simulink model "UBR_SIMULINK_2"  (R2023a)
settings: Solver=VariableStepAuto  StartTime=0.0  StopTime=10  RelTol=1e-3
values from neighbouring files (symbols this model uses):
  g = 9.801    [ubr_3.m]
  vx0 = v0 * cos(theta0)    [ubr_3.m]
  vz0 = v0 * sin(theta0)    [ubr_3.m]
settings Model: Creator=sefab  LastModifiedBy=sefab

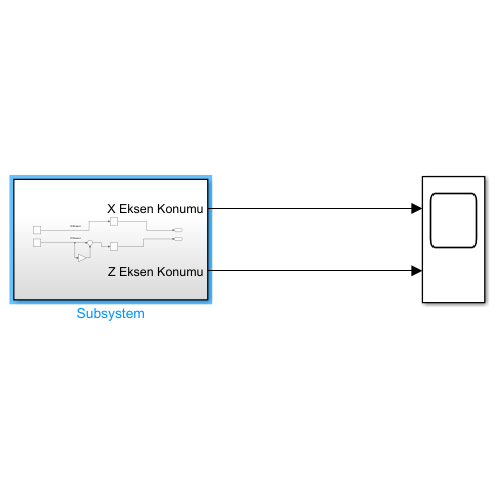
[thumbnail: Simulink's stored preview of the top-level diagram]
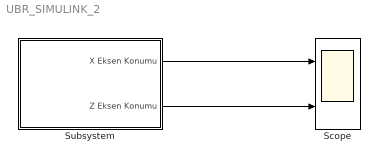
== system UBR_SIMULINK_2 ==
  Scope : Scope  NumInputPorts=2
  Subsystem : Subsystem
  wires:
  Subsystem/1(X Eksen Konumu) -> Scope/1
  Subsystem/2(Z Eksen Konumu) -> Scope/2

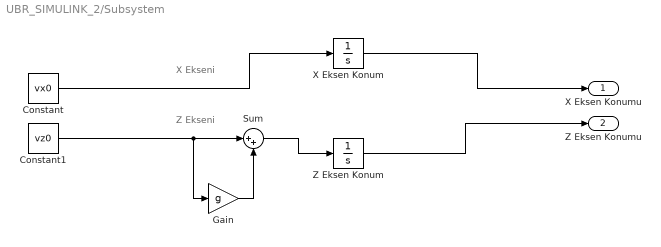
== system UBR_SIMULINK_2/Subsystem ==
  note: Z Ekseni
  note: X Ekseni
  Constant : Constant  Value=vx0
  Constant1 : Constant  Value=vz0
  Gain : Gain  Gain=g
  Sum : Sum  Inputs=|++
  X Eksen Konum : Integrator
  Z Eksen Konum : Integrator
  X Eksen Konumu : Outport
  Z Eksen Konumu : Outport  Port=2
  wires:
  Gain/1 -> Sum/2
  Z Eksen Konum/1 -> Z Eksen Konumu/1
  Sum/1 -> Z Eksen Konum/1
  Constant1/1 -> Gain/1, Sum/1
  X Eksen Konum/1 -> X Eksen Konumu/1
  Constant/1 -> X Eksen Konum/1
